simulink model "fftanalyzeri"  (R2012b)
settings: Solver=ode3  SolverMode=SingleTasking  StartTime=0.0  StopTime=20000  RelTol=1e-3
undefined symbols (not defined in the file or in its folder): pfb_coeff_gen_calc
undefined symbols (not defined in the file): fft_bin_flags_, magphmeanmem_, threshmem_
libraries: xbsIndex_r4 x9073, casper_library_misc x119, casper_library_flow_control x51, casper_library_delays x22, xps_library x10
(part 24 of 74)

== system fftanalyzeri/FIFO64_/FIFO32_1/FIFO16Cir_1/CounterArray2/demux16_ ==
  Chan : Inport
  din : Inport  Port=2
  Demux8_ : Subsystem
  Demux8_1 : Subsystem
  Inverter : xbsIndex_r4/Inverter  en=off  latency=0  dbl_ovrd=off  block_type=inv
  lsb_ui3_ : xbsIndex_r4/Slice  nbits=3  boolean_output=off  mode=Lower Bit Location + Width  bit1=0  base1=MSB of Input  bit0=0  base0=LSB of Input  dbl_ovrd=off  block_type=slice
  msb_b_ : xbsIndex_r4/Slice  nbits=1  boolean_output=on  mode=Upper Bit Location + Width  bit1=0  base1=MSB of Input  bit0=0  base0=LSB of Input  dbl_ovrd=off  block_type=slice
  Out1 : Outport
  Out2 : Outport  Port=2
  Out3 : Outport  Port=3
  Out4 : Outport  Port=4
  Out5 : Outport  Port=5
  Out6 : Outport  Port=6
  Out7 : Outport  Port=7
  Out8 : Outport  Port=8
  Out9 : Outport  Port=9
  Out10 : Outport  Port=10
  Out11 : Outport  Port=11
  Out12 : Outport  Port=12
  Out13 : Outport  Port=13
  Out14 : Outport  Port=14
  Out15 : Outport  Port=15
  Out16 : Outport  Port=16
  wires:
  Demux8_1/1(Out0) -> Out9/1
  Demux8_1/6(Out5) -> Out14/1
  Demux8_/5(Out4) -> Out5/1
  Demux8_/7(Out6) -> Out7/1
  Demux8_1/2(Out1) -> Out10/1
  Demux8_1/3(Out2) -> Out11/1
  Demux8_/4(Out3) -> Out4/1
  Demux8_1/7(Out6) -> Out15/1
  Demux8_1/4(Out3) -> Out12/1
  Demux8_/8(Out7) -> Out8/1
  Demux8_/1(Out0) -> Out1/1
  Demux8_1/5(Out4) -> Out13/1
  Demux8_/6(Out5) -> Out6/1
  Demux8_/2(Out1) -> Out2/1
  Demux8_/3(Out2) -> Out3/1
  Demux8_1/8(Out7) -> Out16/1
  Chan/1 -> msb_b_/1, lsb_ui3_/1
  lsb_ui3_/1 -> Demux8_1/1(Addr), Demux8_/1(Addr)
  msb_b_/1 -> Demux8_1/3(en), Inverter/1
  din/1 -> Demux8_1/2(BitIn), Demux8_/2(BitIn)
  Inverter/1 -> Demux8_/3(en)

== system fftanalyzeri/FIFO64_/FIFO32_1/FIFO16Cir_2/CounterArray1/demux16_ ==
  Chan : Inport
  din : Inport  Port=2
  Demux8_ : Subsystem
  Demux8_1 : Subsystem
  Inverter : xbsIndex_r4/Inverter  en=off  latency=0  dbl_ovrd=off  block_type=inv
  lsb_ui3_ : xbsIndex_r4/Slice  nbits=3  boolean_output=off  mode=Lower Bit Location + Width  bit1=0  base1=MSB of Input  bit0=0  base0=LSB of Input  dbl_ovrd=off  block_type=slice
  msb_b_ : xbsIndex_r4/Slice  nbits=1  boolean_output=on  mode=Upper Bit Location + Width  bit1=0  base1=MSB of Input  bit0=0  base0=LSB of Input  dbl_ovrd=off  block_type=slice
  Out1 : Outport
  Out2 : Outport  Port=2
  Out3 : Outport  Port=3
  Out4 : Outport  Port=4
  Out5 : Outport  Port=5
  Out6 : Outport  Port=6
  Out7 : Outport  Port=7
  Out8 : Outport  Port=8
  Out9 : Outport  Port=9
  Out10 : Outport  Port=10
  Out11 : Outport  Port=11
  Out12 : Outport  Port=12
  Out13 : Outport  Port=13
  Out14 : Outport  Port=14
  Out15 : Outport  Port=15
  Out16 : Outport  Port=16
  wires:
  Demux8_1/1(Out0) -> Out9/1
  Demux8_1/6(Out5) -> Out14/1
  Demux8_/5(Out4) -> Out5/1
  Demux8_/7(Out6) -> Out7/1
  Demux8_1/2(Out1) -> Out10/1
  Demux8_1/3(Out2) -> Out11/1
  Demux8_/4(Out3) -> Out4/1
  Demux8_1/7(Out6) -> Out15/1
  Demux8_1/4(Out3) -> Out12/1
  Demux8_/8(Out7) -> Out8/1
  Demux8_/1(Out0) -> Out1/1
  Demux8_1/5(Out4) -> Out13/1
  Demux8_/6(Out5) -> Out6/1
  Demux8_/2(Out1) -> Out2/1
  Demux8_/3(Out2) -> Out3/1
  Demux8_1/8(Out7) -> Out16/1
  Chan/1 -> msb_b_/1, lsb_ui3_/1
  lsb_ui3_/1 -> Demux8_1/1(Addr), Demux8_/1(Addr)
  msb_b_/1 -> Demux8_1/3(en), Inverter/1
  din/1 -> Demux8_1/2(BitIn), Demux8_/2(BitIn)
  Inverter/1 -> Demux8_/3(en)

== system fftanalyzeri/FIFO64_/FIFO32_1/FIFO16Cir_2/CounterArray2/demux16_ ==
  Chan : Inport
  din : Inport  Port=2
  Demux8_ : Subsystem
  Demux8_1 : Subsystem
  Inverter : xbsIndex_r4/Inverter  en=off  latency=0  dbl_ovrd=off  block_type=inv
  lsb_ui3_ : xbsIndex_r4/Slice  nbits=3  boolean_output=off  mode=Lower Bit Location + Width  bit1=0  base1=MSB of Input  bit0=0  base0=LSB of Input  dbl_ovrd=off  block_type=slice
  msb_b_ : xbsIndex_r4/Slice  nbits=1  boolean_output=on  mode=Upper Bit Location + Width  bit1=0  base1=MSB of Input  bit0=0  base0=LSB of Input  dbl_ovrd=off  block_type=slice
  Out1 : Outport
  Out2 : Outport  Port=2
  Out3 : Outport  Port=3
  Out4 : Outport  Port=4
  Out5 : Outport  Port=5
  Out6 : Outport  Port=6
  Out7 : Outport  Port=7
  Out8 : Outport  Port=8
  Out9 : Outport  Port=9
  Out10 : Outport  Port=10
  Out11 : Outport  Port=11
  Out12 : Outport  Port=12
  Out13 : Outport  Port=13
  Out14 : Outport  Port=14
  Out15 : Outport  Port=15
  Out16 : Outport  Port=16
  wires:
  Demux8_1/1(Out0) -> Out9/1
  Demux8_1/6(Out5) -> Out14/1
  Demux8_/5(Out4) -> Out5/1
  Demux8_/7(Out6) -> Out7/1
  Demux8_1/2(Out1) -> Out10/1
  Demux8_1/3(Out2) -> Out11/1
  Demux8_/4(Out3) -> Out4/1
  Demux8_1/7(Out6) -> Out15/1
  Demux8_1/4(Out3) -> Out12/1
  Demux8_/8(Out7) -> Out8/1
  Demux8_/1(Out0) -> Out1/1
  Demux8_1/5(Out4) -> Out13/1
  Demux8_/6(Out5) -> Out6/1
  Demux8_/2(Out1) -> Out2/1
  Demux8_/3(Out2) -> Out3/1
  Demux8_1/8(Out7) -> Out16/1
  Chan/1 -> msb_b_/1, lsb_ui3_/1
  lsb_ui3_/1 -> Demux8_1/1(Addr), Demux8_/1(Addr)
  msb_b_/1 -> Demux8_1/3(en), Inverter/1
  din/1 -> Demux8_1/2(BitIn), Demux8_/2(BitIn)
  Inverter/1 -> Demux8_/3(en)

== system fftanalyzeri/FIFO64_1/FIFO32_0/FIFO16Cir_1/CounterArray1/demux16_ ==
  Chan : Inport
  din : Inport  Port=2
  Demux8_ : Subsystem
  Demux8_1 : Subsystem
  Inverter : xbsIndex_r4/Inverter  en=off  latency=0  dbl_ovrd=off  block_type=inv
  lsb_ui3_ : xbsIndex_r4/Slice  nbits=3  boolean_output=off  mode=Lower Bit Location + Width  bit1=0  base1=MSB of Input  bit0=0  base0=LSB of Input  dbl_ovrd=off  block_type=slice
  msb_b_ : xbsIndex_r4/Slice  nbits=1  boolean_output=on  mode=Upper Bit Location + Width  bit1=0  base1=MSB of Input  bit0=0  base0=LSB of Input  dbl_ovrd=off  block_type=slice
  Out1 : Outport
  Out2 : Outport  Port=2
  Out3 : Outport  Port=3
  Out4 : Outport  Port=4
  Out5 : Outport  Port=5
  Out6 : Outport  Port=6
  Out7 : Outport  Port=7
  Out8 : Outport  Port=8
  Out9 : Outport  Port=9
  Out10 : Outport  Port=10
  Out11 : Outport  Port=11
  Out12 : Outport  Port=12
  Out13 : Outport  Port=13
  Out14 : Outport  Port=14
  Out15 : Outport  Port=15
  Out16 : Outport  Port=16
  wires:
  Demux8_1/1(Out0) -> Out9/1
  Demux8_1/6(Out5) -> Out14/1
  Demux8_/5(Out4) -> Out5/1
  Demux8_/7(Out6) -> Out7/1
  Demux8_1/2(Out1) -> Out10/1
  Demux8_1/3(Out2) -> Out11/1
  Demux8_/4(Out3) -> Out4/1
  Demux8_1/7(Out6) -> Out15/1
  Demux8_1/4(Out3) -> Out12/1
  Demux8_/8(Out7) -> Out8/1
  Demux8_/1(Out0) -> Out1/1
  Demux8_1/5(Out4) -> Out13/1
  Demux8_/6(Out5) -> Out6/1
  Demux8_/2(Out1) -> Out2/1
  Demux8_/3(Out2) -> Out3/1
  Demux8_1/8(Out7) -> Out16/1
  Chan/1 -> msb_b_/1, lsb_ui3_/1
  lsb_ui3_/1 -> Demux8_1/1(Addr), Demux8_/1(Addr)
  msb_b_/1 -> Demux8_1/3(en), Inverter/1
  din/1 -> Demux8_1/2(BitIn), Demux8_/2(BitIn)
  Inverter/1 -> Demux8_/3(en)

== system fftanalyzeri/FIFO64_1/FIFO32_0/FIFO16Cir_1/CounterArray2/demux16_ ==
  Chan : Inport
  din : Inport  Port=2
  Demux8_ : Subsystem
  Demux8_1 : Subsystem
  Inverter : xbsIndex_r4/Inverter  en=off  latency=0  dbl_ovrd=off  block_type=inv
  lsb_ui3_ : xbsIndex_r4/Slice  nbits=3  boolean_output=off  mode=Lower Bit Location + Width  bit1=0  base1=MSB of Input  bit0=0  base0=LSB of Input  dbl_ovrd=off  block_type=slice
  msb_b_ : xbsIndex_r4/Slice  nbits=1  boolean_output=on  mode=Upper Bit Location + Width  bit1=0  base1=MSB of Input  bit0=0  base0=LSB of Input  dbl_ovrd=off  block_type=slice
  Out1 : Outport
  Out2 : Outport  Port=2
  Out3 : Outport  Port=3
  Out4 : Outport  Port=4
  Out5 : Outport  Port=5
  Out6 : Outport  Port=6
  Out7 : Outport  Port=7
  Out8 : Outport  Port=8
  Out9 : Outport  Port=9
  Out10 : Outport  Port=10
  Out11 : Outport  Port=11
  Out12 : Outport  Port=12
  Out13 : Outport  Port=13
  Out14 : Outport  Port=14
  Out15 : Outport  Port=15
  Out16 : Outport  Port=16
  wires:
  Demux8_1/1(Out0) -> Out9/1
  Demux8_1/6(Out5) -> Out14/1
  Demux8_/5(Out4) -> Out5/1
  Demux8_/7(Out6) -> Out7/1
  Demux8_1/2(Out1) -> Out10/1
  Demux8_1/3(Out2) -> Out11/1
  Demux8_/4(Out3) -> Out4/1
  Demux8_1/7(Out6) -> Out15/1
  Demux8_1/4(Out3) -> Out12/1
  Demux8_/8(Out7) -> Out8/1
  Demux8_/1(Out0) -> Out1/1
  Demux8_1/5(Out4) -> Out13/1
  Demux8_/6(Out5) -> Out6/1
  Demux8_/2(Out1) -> Out2/1
  Demux8_/3(Out2) -> Out3/1
  Demux8_1/8(Out7) -> Out16/1
  Chan/1 -> msb_b_/1, lsb_ui3_/1
  lsb_ui3_/1 -> Demux8_1/1(Addr), Demux8_/1(Addr)
  msb_b_/1 -> Demux8_1/3(en), Inverter/1
  din/1 -> Demux8_1/2(BitIn), Demux8_/2(BitIn)
  Inverter/1 -> Demux8_/3(en)

== system fftanalyzeri/FIFO64_1/FIFO32_0/FIFO16Cir_2/CounterArray1/demux16_ ==
  Chan : Inport
  din : Inport  Port=2
  Demux8_ : Subsystem
  Demux8_1 : Subsystem
  Inverter : xbsIndex_r4/Inverter  en=off  latency=0  dbl_ovrd=off  block_type=inv
  lsb_ui3_ : xbsIndex_r4/Slice  nbits=3  boolean_output=off  mode=Lower Bit Location + Width  bit1=0  base1=MSB of Input  bit0=0  base0=LSB of Input  dbl_ovrd=off  block_type=slice
  msb_b_ : xbsIndex_r4/Slice  nbits=1  boolean_output=on  mode=Upper Bit Location + Width  bit1=0  base1=MSB of Input  bit0=0  base0=LSB of Input  dbl_ovrd=off  block_type=slice
  Out1 : Outport
  Out2 : Outport  Port=2
  Out3 : Outport  Port=3
  Out4 : Outport  Port=4
  Out5 : Outport  Port=5
  Out6 : Outport  Port=6
  Out7 : Outport  Port=7
  Out8 : Outport  Port=8
  Out9 : Outport  Port=9
  Out10 : Outport  Port=10
  Out11 : Outport  Port=11
  Out12 : Outport  Port=12
  Out13 : Outport  Port=13
  Out14 : Outport  Port=14
  Out15 : Outport  Port=15
  Out16 : Outport  Port=16
  wires:
  Demux8_1/1(Out0) -> Out9/1
  Demux8_1/6(Out5) -> Out14/1
  Demux8_/5(Out4) -> Out5/1
  Demux8_/7(Out6) -> Out7/1
  Demux8_1/2(Out1) -> Out10/1
  Demux8_1/3(Out2) -> Out11/1
  Demux8_/4(Out3) -> Out4/1
  Demux8_1/7(Out6) -> Out15/1
  Demux8_1/4(Out3) -> Out12/1
  Demux8_/8(Out7) -> Out8/1
  Demux8_/1(Out0) -> Out1/1
  Demux8_1/5(Out4) -> Out13/1
  Demux8_/6(Out5) -> Out6/1
  Demux8_/2(Out1) -> Out2/1
  Demux8_/3(Out2) -> Out3/1
  Demux8_1/8(Out7) -> Out16/1
  Chan/1 -> msb_b_/1, lsb_ui3_/1
  lsb_ui3_/1 -> Demux8_1/1(Addr), Demux8_/1(Addr)
  msb_b_/1 -> Demux8_1/3(en), Inverter/1
  din/1 -> Demux8_1/2(BitIn), Demux8_/2(BitIn)
  Inverter/1 -> Demux8_/3(en)

== system fftanalyzeri/FIFO64_1/FIFO32_0/FIFO16Cir_2/CounterArray2/demux16_ ==
  Chan : Inport
  din : Inport  Port=2
  Demux8_ : Subsystem
  Demux8_1 : Subsystem
  Inverter : xbsIndex_r4/Inverter  en=off  latency=0  dbl_ovrd=off  block_type=inv
  lsb_ui3_ : xbsIndex_r4/Slice  nbits=3  boolean_output=off  mode=Lower Bit Location + Width  bit1=0  base1=MSB of Input  bit0=0  base0=LSB of Input  dbl_ovrd=off  block_type=slice
  msb_b_ : xbsIndex_r4/Slice  nbits=1  boolean_output=on  mode=Upper Bit Location + Width  bit1=0  base1=MSB of Input  bit0=0  base0=LSB of Input  dbl_ovrd=off  block_type=slice
  Out1 : Outport
  Out2 : Outport  Port=2
  Out3 : Outport  Port=3
  Out4 : Outport  Port=4
  Out5 : Outport  Port=5
  Out6 : Outport  Port=6
  Out7 : Outport  Port=7
  Out8 : Outport  Port=8
  Out9 : Outport  Port=9
  Out10 : Outport  Port=10
  Out11 : Outport  Port=11
  Out12 : Outport  Port=12
  Out13 : Outport  Port=13
  Out14 : Outport  Port=14
  Out15 : Outport  Port=15
  Out16 : Outport  Port=16
  wires:
  Demux8_1/1(Out0) -> Out9/1
  Demux8_1/6(Out5) -> Out14/1
  Demux8_/5(Out4) -> Out5/1
  Demux8_/7(Out6) -> Out7/1
  Demux8_1/2(Out1) -> Out10/1
  Demux8_1/3(Out2) -> Out11/1
  Demux8_/4(Out3) -> Out4/1
  Demux8_1/7(Out6) -> Out15/1
  Demux8_1/4(Out3) -> Out12/1
  Demux8_/8(Out7) -> Out8/1
  Demux8_/1(Out0) -> Out1/1
  Demux8_1/5(Out4) -> Out13/1
  Demux8_/6(Out5) -> Out6/1
  Demux8_/2(Out1) -> Out2/1
  Demux8_/3(Out2) -> Out3/1
  Demux8_1/8(Out7) -> Out16/1
  Chan/1 -> msb_b_/1, lsb_ui3_/1
  lsb_ui3_/1 -> Demux8_1/1(Addr), Demux8_/1(Addr)
  msb_b_/1 -> Demux8_1/3(en), Inverter/1
  din/1 -> Demux8_1/2(BitIn), Demux8_/2(BitIn)
  Inverter/1 -> Demux8_/3(en)

== system fftanalyzeri/FIFO64_1/FIFO32_1/FIFO16Cir_1/CounterArray1/demux16_ ==
  Chan : Inport
  din : Inport  Port=2
  Demux8_ : Subsystem
  Demux8_1 : Subsystem
  Inverter : xbsIndex_r4/Inverter  en=off  latency=0  dbl_ovrd=off  block_type=inv
  lsb_ui3_ : xbsIndex_r4/Slice  nbits=3  boolean_output=off  mode=Lower Bit Location + Width  bit1=0  base1=MSB of Input  bit0=0  base0=LSB of Input  dbl_ovrd=off  block_type=slice
  msb_b_ : xbsIndex_r4/Slice  nbits=1  boolean_output=on  mode=Upper Bit Location + Width  bit1=0  base1=MSB of Input  bit0=0  base0=LSB of Input  dbl_ovrd=off  block_type=slice
  Out1 : Outport
  Out2 : Outport  Port=2
  Out3 : Outport  Port=3
  Out4 : Outport  Port=4
  Out5 : Outport  Port=5
  Out6 : Outport  Port=6
  Out7 : Outport  Port=7
  Out8 : Outport  Port=8
  Out9 : Outport  Port=9
  Out10 : Outport  Port=10
  Out11 : Outport  Port=11
  Out12 : Outport  Port=12
  Out13 : Outport  Port=13
  Out14 : Outport  Port=14
  Out15 : Outport  Port=15
  Out16 : Outport  Port=16
  wires:
  Demux8_1/1(Out0) -> Out9/1
  Demux8_1/6(Out5) -> Out14/1
  Demux8_/5(Out4) -> Out5/1
  Demux8_/7(Out6) -> Out7/1
  Demux8_1/2(Out1) -> Out10/1
  Demux8_1/3(Out2) -> Out11/1
  Demux8_/4(Out3) -> Out4/1
  Demux8_1/7(Out6) -> Out15/1
  Demux8_1/4(Out3) -> Out12/1
  Demux8_/8(Out7) -> Out8/1
  Demux8_/1(Out0) -> Out1/1
  Demux8_1/5(Out4) -> Out13/1
  Demux8_/6(Out5) -> Out6/1
  Demux8_/2(Out1) -> Out2/1
  Demux8_/3(Out2) -> Out3/1
  Demux8_1/8(Out7) -> Out16/1
  Chan/1 -> msb_b_/1, lsb_ui3_/1
  lsb_ui3_/1 -> Demux8_1/1(Addr), Demux8_/1(Addr)
  msb_b_/1 -> Demux8_1/3(en), Inverter/1
  din/1 -> Demux8_1/2(BitIn), Demux8_/2(BitIn)
  Inverter/1 -> Demux8_/3(en)

== system fftanalyzeri/FIFO64_1/FIFO32_1/FIFO16Cir_1/CounterArray2/demux16_ ==
  Chan : Inport
  din : Inport  Port=2
  Demux8_ : Subsystem
  Demux8_1 : Subsystem
  Inverter : xbsIndex_r4/Inverter  en=off  latency=0  dbl_ovrd=off  block_type=inv
  lsb_ui3_ : xbsIndex_r4/Slice  nbits=3  boolean_output=off  mode=Lower Bit Location + Width  bit1=0  base1=MSB of Input  bit0=0  base0=LSB of Input  dbl_ovrd=off  block_type=slice
  msb_b_ : xbsIndex_r4/Slice  nbits=1  boolean_output=on  mode=Upper Bit Location + Width  bit1=0  base1=MSB of Input  bit0=0  base0=LSB of Input  dbl_ovrd=off  block_type=slice
  Out1 : Outport
  Out2 : Outport  Port=2
  Out3 : Outport  Port=3
  Out4 : Outport  Port=4
  Out5 : Outport  Port=5
  Out6 : Outport  Port=6
  Out7 : Outport  Port=7
  Out8 : Outport  Port=8
  Out9 : Outport  Port=9
  Out10 : Outport  Port=10
  Out11 : Outport  Port=11
  Out12 : Outport  Port=12
  Out13 : Outport  Port=13
  Out14 : Outport  Port=14
  Out15 : Outport  Port=15
  Out16 : Outport  Port=16
  wires:
  Demux8_1/1(Out0) -> Out9/1
  Demux8_1/6(Out5) -> Out14/1
  Demux8_/5(Out4) -> Out5/1
  Demux8_/7(Out6) -> Out7/1
  Demux8_1/2(Out1) -> Out10/1
  Demux8_1/3(Out2) -> Out11/1
  Demux8_/4(Out3) -> Out4/1
  Demux8_1/7(Out6) -> Out15/1
  Demux8_1/4(Out3) -> Out12/1
  Demux8_/8(Out7) -> Out8/1
  Demux8_/1(Out0) -> Out1/1
  Demux8_1/5(Out4) -> Out13/1
  Demux8_/6(Out5) -> Out6/1
  Demux8_/2(Out1) -> Out2/1
  Demux8_/3(Out2) -> Out3/1
  Demux8_1/8(Out7) -> Out16/1
  Chan/1 -> msb_b_/1, lsb_ui3_/1
  lsb_ui3_/1 -> Demux8_1/1(Addr), Demux8_/1(Addr)
  msb_b_/1 -> Demux8_1/3(en), Inverter/1
  din/1 -> Demux8_1/2(BitIn), Demux8_/2(BitIn)
  Inverter/1 -> Demux8_/3(en)

== system fftanalyzeri/FIFO64_1/FIFO32_1/FIFO16Cir_2/CounterArray1/demux16_ ==
  Chan : Inport
  din : Inport  Port=2
  Demux8_ : Subsystem
  Demux8_1 : Subsystem
  Inverter : xbsIndex_r4/Inverter  en=off  latency=0  dbl_ovrd=off  block_type=inv
  lsb_ui3_ : xbsIndex_r4/Slice  nbits=3  boolean_output=off  mode=Lower Bit Location + Width  bit1=0  base1=MSB of Input  bit0=0  base0=LSB of Input  dbl_ovrd=off  block_type=slice
  msb_b_ : xbsIndex_r4/Slice  nbits=1  boolean_output=on  mode=Upper Bit Location + Width  bit1=0  base1=MSB of Input  bit0=0  base0=LSB of Input  dbl_ovrd=off  block_type=slice
  Out1 : Outport
  Out2 : Outport  Port=2
  Out3 : Outport  Port=3
  Out4 : Outport  Port=4
  Out5 : Outport  Port=5
  Out6 : Outport  Port=6
  Out7 : Outport  Port=7
  Out8 : Outport  Port=8
  Out9 : Outport  Port=9
  Out10 : Outport  Port=10
  Out11 : Outport  Port=11
  Out12 : Outport  Port=12
  Out13 : Outport  Port=13
  Out14 : Outport  Port=14
  Out15 : Outport  Port=15
  Out16 : Outport  Port=16
  wires:
  Demux8_1/1(Out0) -> Out9/1
  Demux8_1/6(Out5) -> Out14/1
  Demux8_/5(Out4) -> Out5/1
  Demux8_/7(Out6) -> Out7/1
  Demux8_1/2(Out1) -> Out10/1
  Demux8_1/3(Out2) -> Out11/1
  Demux8_/4(Out3) -> Out4/1
  Demux8_1/7(Out6) -> Out15/1
  Demux8_1/4(Out3) -> Out12/1
  Demux8_/8(Out7) -> Out8/1
  Demux8_/1(Out0) -> Out1/1
  Demux8_1/5(Out4) -> Out13/1
  Demux8_/6(Out5) -> Out6/1
  Demux8_/2(Out1) -> Out2/1
  Demux8_/3(Out2) -> Out3/1
  Demux8_1/8(Out7) -> Out16/1
  Chan/1 -> msb_b_/1, lsb_ui3_/1
  lsb_ui3_/1 -> Demux8_1/1(Addr), Demux8_/1(Addr)
  msb_b_/1 -> Demux8_1/3(en), Inverter/1
  din/1 -> Demux8_1/2(BitIn), Demux8_/2(BitIn)
  Inverter/1 -> Demux8_/3(en)

== system fftanalyzeri/FIFO64_1/FIFO32_1/FIFO16Cir_2/CounterArray2/demux16_ ==
  Chan : Inport
  din : Inport  Port=2
  Demux8_ : Subsystem
  Demux8_1 : Subsystem
  Inverter : xbsIndex_r4/Inverter  en=off  latency=0  dbl_ovrd=off  block_type=inv
  lsb_ui3_ : xbsIndex_r4/Slice  nbits=3  boolean_output=off  mode=Lower Bit Location + Width  bit1=0  base1=MSB of Input  bit0=0  base0=LSB of Input  dbl_ovrd=off  block_type=slice
  msb_b_ : xbsIndex_r4/Slice  nbits=1  boolean_output=on  mode=Upper Bit Location + Width  bit1=0  base1=MSB of Input  bit0=0  base0=LSB of Input  dbl_ovrd=off  block_type=slice
  Out1 : Outport
  Out2 : Outport  Port=2
  Out3 : Outport  Port=3
  Out4 : Outport  Port=4
  Out5 : Outport  Port=5
  Out6 : Outport  Port=6
  Out7 : Outport  Port=7
  Out8 : Outport  Port=8
  Out9 : Outport  Port=9
  Out10 : Outport  Port=10
  Out11 : Outport  Port=11
  Out12 : Outport  Port=12
  Out13 : Outport  Port=13
  Out14 : Outport  Port=14
  Out15 : Outport  Port=15
  Out16 : Outport  Port=16
  wires:
  Demux8_1/1(Out0) -> Out9/1
  Demux8_1/6(Out5) -> Out14/1
  Demux8_/5(Out4) -> Out5/1
  Demux8_/7(Out6) -> Out7/1
  Demux8_1/2(Out1) -> Out10/1
  Demux8_1/3(Out2) -> Out11/1
  Demux8_/4(Out3) -> Out4/1
  Demux8_1/7(Out6) -> Out15/1
  Demux8_1/4(Out3) -> Out12/1
  Demux8_/8(Out7) -> Out8/1
  Demux8_/1(Out0) -> Out1/1
  Demux8_1/5(Out4) -> Out13/1
  Demux8_/6(Out5) -> Out6/1
  Demux8_/2(Out1) -> Out2/1
  Demux8_/3(Out2) -> Out3/1
  Demux8_1/8(Out7) -> Out16/1
  Chan/1 -> msb_b_/1, lsb_ui3_/1
  lsb_ui3_/1 -> Demux8_1/1(Addr), Demux8_/1(Addr)
  msb_b_/1 -> Demux8_1/3(en), Inverter/1
  din/1 -> Demux8_1/2(BitIn), Demux8_/2(BitIn)
  Inverter/1 -> Demux8_/3(en)

== system fftanalyzeri/FIFO64_2/FIFO32_0/FIFO16Cir_1/CounterArray1/demux16_ ==
  Chan : Inport
  din : Inport  Port=2
  Demux8_ : Subsystem
  Demux8_1 : Subsystem
  Inverter : xbsIndex_r4/Inverter  en=off  latency=0  dbl_ovrd=off  block_type=inv
  lsb_ui3_ : xbsIndex_r4/Slice  nbits=3  boolean_output=off  mode=Lower Bit Location + Width  bit1=0  base1=MSB of Input  bit0=0  base0=LSB of Input  dbl_ovrd=off  block_type=slice
  msb_b_ : xbsIndex_r4/Slice  nbits=1  boolean_output=on  mode=Upper Bit Location + Width  bit1=0  base1=MSB of Input  bit0=0  base0=LSB of Input  dbl_ovrd=off  block_type=slice
  Out1 : Outport
  Out2 : Outport  Port=2
  Out3 : Outport  Port=3
  Out4 : Outport  Port=4
  Out5 : Outport  Port=5
  Out6 : Outport  Port=6
  Out7 : Outport  Port=7
  Out8 : Outport  Port=8
  Out9 : Outport  Port=9
  Out10 : Outport  Port=10
  Out11 : Outport  Port=11
  Out12 : Outport  Port=12
  Out13 : Outport  Port=13
  Out14 : Outport  Port=14
  Out15 : Outport  Port=15
  Out16 : Outport  Port=16
  wires:
  Demux8_1/1(Out0) -> Out9/1
  Demux8_1/6(Out5) -> Out14/1
  Demux8_/5(Out4) -> Out5/1
  Demux8_/7(Out6) -> Out7/1
  Demux8_1/2(Out1) -> Out10/1
  Demux8_1/3(Out2) -> Out11/1
  Demux8_/4(Out3) -> Out4/1
  Demux8_1/7(Out6) -> Out15/1
  Demux8_1/4(Out3) -> Out12/1
  Demux8_/8(Out7) -> Out8/1
  Demux8_/1(Out0) -> Out1/1
  Demux8_1/5(Out4) -> Out13/1
  Demux8_/6(Out5) -> Out6/1
  Demux8_/2(Out1) -> Out2/1
  Demux8_/3(Out2) -> Out3/1
  Demux8_1/8(Out7) -> Out16/1
  Chan/1 -> msb_b_/1, lsb_ui3_/1
  lsb_ui3_/1 -> Demux8_1/1(Addr), Demux8_/1(Addr)
  msb_b_/1 -> Demux8_1/3(en), Inverter/1
  din/1 -> Demux8_1/2(BitIn), Demux8_/2(BitIn)
  Inverter/1 -> Demux8_/3(en)

== system fftanalyzeri/FIFO64_2/FIFO32_0/FIFO16Cir_1/CounterArray2/demux16_ ==
  Chan : Inport
  din : Inport  Port=2
  Demux8_ : Subsystem
  Demux8_1 : Subsystem
  Inverter : xbsIndex_r4/Inverter  en=off  latency=0  dbl_ovrd=off  block_type=inv
  lsb_ui3_ : xbsIndex_r4/Slice  nbits=3  boolean_output=off  mode=Lower Bit Location + Width  bit1=0  base1=MSB of Input  bit0=0  base0=LSB of Input  dbl_ovrd=off  block_type=slice
  msb_b_ : xbsIndex_r4/Slice  nbits=1  boolean_output=on  mode=Upper Bit Location + Width  bit1=0  base1=MSB of Input  bit0=0  base0=LSB of Input  dbl_ovrd=off  block_type=slice
  Out1 : Outport
  Out2 : Outport  Port=2
  Out3 : Outport  Port=3
  Out4 : Outport  Port=4
  Out5 : Outport  Port=5
  Out6 : Outport  Port=6
  Out7 : Outport  Port=7
  Out8 : Outport  Port=8
  Out9 : Outport  Port=9
  Out10 : Outport  Port=10
  Out11 : Outport  Port=11
  Out12 : Outport  Port=12
  Out13 : Outport  Port=13
  Out14 : Outport  Port=14
  Out15 : Outport  Port=15
  Out16 : Outport  Port=16
  wires:
  Demux8_1/1(Out0) -> Out9/1
  Demux8_1/6(Out5) -> Out14/1
  Demux8_/5(Out4) -> Out5/1
  Demux8_/7(Out6) -> Out7/1
  Demux8_1/2(Out1) -> Out10/1
  Demux8_1/3(Out2) -> Out11/1
  Demux8_/4(Out3) -> Out4/1
  Demux8_1/7(Out6) -> Out15/1
  Demux8_1/4(Out3) -> Out12/1
  Demux8_/8(Out7) -> Out8/1
  Demux8_/1(Out0) -> Out1/1
  Demux8_1/5(Out4) -> Out13/1
  Demux8_/6(Out5) -> Out6/1
  Demux8_/2(Out1) -> Out2/1
  Demux8_/3(Out2) -> Out3/1
  Demux8_1/8(Out7) -> Out16/1
  Chan/1 -> msb_b_/1, lsb_ui3_/1
  lsb_ui3_/1 -> Demux8_1/1(Addr), Demux8_/1(Addr)
  msb_b_/1 -> Demux8_1/3(en), Inverter/1
  din/1 -> Demux8_1/2(BitIn), Demux8_/2(BitIn)
  Inverter/1 -> Demux8_/3(en)

== system fftanalyzeri/FIFO64_2/FIFO32_0/FIFO16Cir_2/CounterArray1/demux16_ ==
  Chan : Inport
  din : Inport  Port=2
  Demux8_ : Subsystem
  Demux8_1 : Subsystem
  Inverter : xbsIndex_r4/Inverter  en=off  latency=0  dbl_ovrd=off  block_type=inv
  lsb_ui3_ : xbsIndex_r4/Slice  nbits=3  boolean_output=off  mode=Lower Bit Location + Width  bit1=0  base1=MSB of Input  bit0=0  base0=LSB of Input  dbl_ovrd=off  block_type=slice
  msb_b_ : xbsIndex_r4/Slice  nbits=1  boolean_output=on  mode=Upper Bit Location + Width  bit1=0  base1=MSB of Input  bit0=0  base0=LSB of Input  dbl_ovrd=off  block_type=slice
  Out1 : Outport
  Out2 : Outport  Port=2
  Out3 : Outport  Port=3
  Out4 : Outport  Port=4
  Out5 : Outport  Port=5
  Out6 : Outport  Port=6
  Out7 : Outport  Port=7
  Out8 : Outport  Port=8
  Out9 : Outport  Port=9
  Out10 : Outport  Port=10
  Out11 : Outport  Port=11
  Out12 : Outport  Port=12
  Out13 : Outport  Port=13
  Out14 : Outport  Port=14
  Out15 : Outport  Port=15
  Out16 : Outport  Port=16
  wires:
  Demux8_1/1(Out0) -> Out9/1
  Demux8_1/6(Out5) -> Out14/1
  Demux8_/5(Out4) -> Out5/1
  Demux8_/7(Out6) -> Out7/1
  Demux8_1/2(Out1) -> Out10/1
  Demux8_1/3(Out2) -> Out11/1
  Demux8_/4(Out3) -> Out4/1
  Demux8_1/7(Out6) -> Out15/1
  Demux8_1/4(Out3) -> Out12/1
  Demux8_/8(Out7) -> Out8/1
  Demux8_/1(Out0) -> Out1/1
  Demux8_1/5(Out4) -> Out13/1
  Demux8_/6(Out5) -> Out6/1
  Demux8_/2(Out1) -> Out2/1
  Demux8_/3(Out2) -> Out3/1
  Demux8_1/8(Out7) -> Out16/1
  Chan/1 -> msb_b_/1, lsb_ui3_/1
  lsb_ui3_/1 -> Demux8_1/1(Addr), Demux8_/1(Addr)
  msb_b_/1 -> Demux8_1/3(en), Inverter/1
  din/1 -> Demux8_1/2(BitIn), Demux8_/2(BitIn)
  Inverter/1 -> Demux8_/3(en)

== system fftanalyzeri/FIFO64_2/FIFO32_0/FIFO16Cir_2/CounterArray2/demux16_ ==
  Chan : Inport
  din : Inport  Port=2
  Demux8_ : Subsystem
  Demux8_1 : Subsystem
  Inverter : xbsIndex_r4/Inverter  en=off  latency=0  dbl_ovrd=off  block_type=inv
  lsb_ui3_ : xbsIndex_r4/Slice  nbits=3  boolean_output=off  mode=Lower Bit Location + Width  bit1=0  base1=MSB of Input  bit0=0  base0=LSB of Input  dbl_ovrd=off  block_type=slice
  msb_b_ : xbsIndex_r4/Slice  nbits=1  boolean_output=on  mode=Upper Bit Location + Width  bit1=0  base1=MSB of Input  bit0=0  base0=LSB of Input  dbl_ovrd=off  block_type=slice
  Out1 : Outport
  Out2 : Outport  Port=2
  Out3 : Outport  Port=3
  Out4 : Outport  Port=4
  Out5 : Outport  Port=5
  Out6 : Outport  Port=6
  Out7 : Outport  Port=7
  Out8 : Outport  Port=8
  Out9 : Outport  Port=9
  Out10 : Outport  Port=10
  Out11 : Outport  Port=11
  Out12 : Outport  Port=12
  Out13 : Outport  Port=13
  Out14 : Outport  Port=14
  Out15 : Outport  Port=15
  Out16 : Outport  Port=16
  wires:
  Demux8_1/1(Out0) -> Out9/1
  Demux8_1/6(Out5) -> Out14/1
  Demux8_/5(Out4) -> Out5/1
  Demux8_/7(Out6) -> Out7/1
  Demux8_1/2(Out1) -> Out10/1
  Demux8_1/3(Out2) -> Out11/1
  Demux8_/4(Out3) -> Out4/1
  Demux8_1/7(Out6) -> Out15/1
  Demux8_1/4(Out3) -> Out12/1
  Demux8_/8(Out7) -> Out8/1
  Demux8_/1(Out0) -> Out1/1
  Demux8_1/5(Out4) -> Out13/1
  Demux8_/6(Out5) -> Out6/1
  Demux8_/2(Out1) -> Out2/1
  Demux8_/3(Out2) -> Out3/1
  Demux8_1/8(Out7) -> Out16/1
  Chan/1 -> msb_b_/1, lsb_ui3_/1
  lsb_ui3_/1 -> Demux8_1/1(Addr), Demux8_/1(Addr)
  msb_b_/1 -> Demux8_1/3(en), Inverter/1
  din/1 -> Demux8_1/2(BitIn), Demux8_/2(BitIn)
  Inverter/1 -> Demux8_/3(en)

== system fftanalyzeri/FIFO64_2/FIFO32_1/FIFO16Cir_1/CounterArray1/demux16_ ==
  Chan : Inport
  din : Inport  Port=2
  Demux8_ : Subsystem
  Demux8_1 : Subsystem
  Inverter : xbsIndex_r4/Inverter  en=off  latency=0  dbl_ovrd=off  block_type=inv
  lsb_ui3_ : xbsIndex_r4/Slice  nbits=3  boolean_output=off  mode=Lower Bit Location + Width  bit1=0  base1=MSB of Input  bit0=0  base0=LSB of Input  dbl_ovrd=off  block_type=slice
  msb_b_ : xbsIndex_r4/Slice  nbits=1  boolean_output=on  mode=Upper Bit Location + Width  bit1=0  base1=MSB of Input  bit0=0  base0=LSB of Input  dbl_ovrd=off  block_type=slice
  Out1 : Outport
  Out2 : Outport  Port=2
  Out3 : Outport  Port=3
  Out4 : Outport  Port=4
  Out5 : Outport  Port=5
  Out6 : Outport  Port=6
  Out7 : Outport  Port=7
  Out8 : Outport  Port=8
  Out9 : Outport  Port=9
  Out10 : Outport  Port=10
  Out11 : Outport  Port=11
  Out12 : Outport  Port=12
  Out13 : Outport  Port=13
  Out14 : Outport  Port=14
  Out15 : Outport  Port=15
  Out16 : Outport  Port=16
  wires:
  Demux8_1/1(Out0) -> Out9/1
  Demux8_1/6(Out5) -> Out14/1
  Demux8_/5(Out4) -> Out5/1
  Demux8_/7(Out6) -> Out7/1
  Demux8_1/2(Out1) -> Out10/1
  Demux8_1/3(Out2) -> Out11/1
  Demux8_/4(Out3) -> Out4/1
  Demux8_1/7(Out6) -> Out15/1
  Demux8_1/4(Out3) -> Out12/1
  Demux8_/8(Out7) -> Out8/1
  Demux8_/1(Out0) -> Out1/1
  Demux8_1/5(Out4) -> Out13/1
  Demux8_/6(Out5) -> Out6/1
  Demux8_/2(Out1) -> Out2/1
  Demux8_/3(Out2) -> Out3/1
  Demux8_1/8(Out7) -> Out16/1
  Chan/1 -> msb_b_/1, lsb_ui3_/1
  lsb_ui3_/1 -> Demux8_1/1(Addr), Demux8_/1(Addr)
  msb_b_/1 -> Demux8_1/3(en), Inverter/1
  din/1 -> Demux8_1/2(BitIn), Demux8_/2(BitIn)
  Inverter/1 -> Demux8_/3(en)

== system fftanalyzeri/FIFO64_2/FIFO32_1/FIFO16Cir_1/CounterArray2/demux16_ ==
  Chan : Inport
  din : Inport  Port=2
  Demux8_ : Subsystem
  Demux8_1 : Subsystem
  Inverter : xbsIndex_r4/Inverter  en=off  latency=0  dbl_ovrd=off  block_type=inv
  lsb_ui3_ : xbsIndex_r4/Slice  nbits=3  boolean_output=off  mode=Lower Bit Location + Width  bit1=0  base1=MSB of Input  bit0=0  base0=LSB of Input  dbl_ovrd=off  block_type=slice
  msb_b_ : xbsIndex_r4/Slice  nbits=1  boolean_output=on  mode=Upper Bit Location + Width  bit1=0  base1=MSB of Input  bit0=0  base0=LSB of Input  dbl_ovrd=off  block_type=slice
  Out1 : Outport
  Out2 : Outport  Port=2
  Out3 : Outport  Port=3
  Out4 : Outport  Port=4
  Out5 : Outport  Port=5
  Out6 : Outport  Port=6
  Out7 : Outport  Port=7
  Out8 : Outport  Port=8
  Out9 : Outport  Port=9
  Out10 : Outport  Port=10
  Out11 : Outport  Port=11
  Out12 : Outport  Port=12
  Out13 : Outport  Port=13
  Out14 : Outport  Port=14
  Out15 : Outport  Port=15
  Out16 : Outport  Port=16
  wires:
  Demux8_1/1(Out0) -> Out9/1
  Demux8_1/6(Out5) -> Out14/1
  Demux8_/5(Out4) -> Out5/1
  Demux8_/7(Out6) -> Out7/1
  Demux8_1/2(Out1) -> Out10/1
  Demux8_1/3(Out2) -> Out11/1
  Demux8_/4(Out3) -> Out4/1
  Demux8_1/7(Out6) -> Out15/1
  Demux8_1/4(Out3) -> Out12/1
  Demux8_/8(Out7) -> Out8/1
  Demux8_/1(Out0) -> Out1/1
  Demux8_1/5(Out4) -> Out13/1
  Demux8_/6(Out5) -> Out6/1
  Demux8_/2(Out1) -> Out2/1
  Demux8_/3(Out2) -> Out3/1
  Demux8_1/8(Out7) -> Out16/1
  Chan/1 -> msb_b_/1, lsb_ui3_/1
  lsb_ui3_/1 -> Demux8_1/1(Addr), Demux8_/1(Addr)
  msb_b_/1 -> Demux8_1/3(en), Inverter/1
  din/1 -> Demux8_1/2(BitIn), Demux8_/2(BitIn)
  Inverter/1 -> Demux8_/3(en)

== system fftanalyzeri/FIFO64_2/FIFO32_1/FIFO16Cir_2/CounterArray1/demux16_ ==
  Chan : Inport
  din : Inport  Port=2
  Demux8_ : Subsystem
  Demux8_1 : Subsystem
  Inverter : xbsIndex_r4/Inverter  en=off  latency=0  dbl_ovrd=off  block_type=inv
  lsb_ui3_ : xbsIndex_r4/Slice  nbits=3  boolean_output=off  mode=Lower Bit Location + Width  bit1=0  base1=MSB of Input  bit0=0  base0=LSB of Input  dbl_ovrd=off  block_type=slice
  msb_b_ : xbsIndex_r4/Slice  nbits=1  boolean_output=on  mode=Upper Bit Location + Width  bit1=0  base1=MSB of Input  bit0=0  base0=LSB of Input  dbl_ovrd=off  block_type=slice
  Out1 : Outport
  Out2 : Outport  Port=2
  Out3 : Outport  Port=3
  Out4 : Outport  Port=4
  Out5 : Outport  Port=5
  Out6 : Outport  Port=6
  Out7 : Outport  Port=7
  Out8 : Outport  Port=8
  Out9 : Outport  Port=9
  Out10 : Outport  Port=10
  Out11 : Outport  Port=11
  Out12 : Outport  Port=12
  Out13 : Outport  Port=13
  Out14 : Outport  Port=14
  Out15 : Outport  Port=15
  Out16 : Outport  Port=16
  wires:
  Demux8_1/1(Out0) -> Out9/1
  Demux8_1/6(Out5) -> Out14/1
  Demux8_/5(Out4) -> Out5/1
  Demux8_/7(Out6) -> Out7/1
  Demux8_1/2(Out1) -> Out10/1
  Demux8_1/3(Out2) -> Out11/1
  Demux8_/4(Out3) -> Out4/1
  Demux8_1/7(Out6) -> Out15/1
  Demux8_1/4(Out3) -> Out12/1
  Demux8_/8(Out7) -> Out8/1
  Demux8_/1(Out0) -> Out1/1
  Demux8_1/5(Out4) -> Out13/1
  Demux8_/6(Out5) -> Out6/1
  Demux8_/2(Out1) -> Out2/1
  Demux8_/3(Out2) -> Out3/1
  Demux8_1/8(Out7) -> Out16/1
  Chan/1 -> msb_b_/1, lsb_ui3_/1
  lsb_ui3_/1 -> Demux8_1/1(Addr), Demux8_/1(Addr)
  msb_b_/1 -> Demux8_1/3(en), Inverter/1
  din/1 -> Demux8_1/2(BitIn), Demux8_/2(BitIn)
  Inverter/1 -> Demux8_/3(en)

== system fftanalyzeri/FIFO64_2/FIFO32_1/FIFO16Cir_2/CounterArray2/demux16_ ==
  Chan : Inport
  din : Inport  Port=2
  Demux8_ : Subsystem
  Demux8_1 : Subsystem
  Inverter : xbsIndex_r4/Inverter  en=off  latency=0  dbl_ovrd=off  block_type=inv
  lsb_ui3_ : xbsIndex_r4/Slice  nbits=3  boolean_output=off  mode=Lower Bit Location + Width  bit1=0  base1=MSB of Input  bit0=0  base0=LSB of Input  dbl_ovrd=off  block_type=slice
  msb_b_ : xbsIndex_r4/Slice  nbits=1  boolean_output=on  mode=Upper Bit Location + Width  bit1=0  base1=MSB of Input  bit0=0  base0=LSB of Input  dbl_ovrd=off  block_type=slice
  Out1 : Outport
  Out2 : Outport  Port=2
  Out3 : Outport  Port=3
  Out4 : Outport  Port=4
  Out5 : Outport  Port=5
  Out6 : Outport  Port=6
  Out7 : Outport  Port=7
  Out8 : Outport  Port=8
  Out9 : Outport  Port=9
  Out10 : Outport  Port=10
  Out11 : Outport  Port=11
  Out12 : Outport  Port=12
  Out13 : Outport  Port=13
  Out14 : Outport  Port=14
  Out15 : Outport  Port=15
  Out16 : Outport  Port=16
  wires:
  Demux8_1/1(Out0) -> Out9/1
  Demux8_1/6(Out5) -> Out14/1
  Demux8_/5(Out4) -> Out5/1
  Demux8_/7(Out6) -> Out7/1
  Demux8_1/2(Out1) -> Out10/1
  Demux8_1/3(Out2) -> Out11/1
  Demux8_/4(Out3) -> Out4/1
  Demux8_1/7(Out6) -> Out15/1
  Demux8_1/4(Out3) -> Out12/1
  Demux8_/8(Out7) -> Out8/1
  Demux8_/1(Out0) -> Out1/1
  Demux8_1/5(Out4) -> Out13/1
  Demux8_/6(Out5) -> Out6/1
  Demux8_/2(Out1) -> Out2/1
  Demux8_/3(Out2) -> Out3/1
  Demux8_1/8(Out7) -> Out16/1
  Chan/1 -> msb_b_/1, lsb_ui3_/1
  lsb_ui3_/1 -> Demux8_1/1(Addr), Demux8_/1(Addr)
  msb_b_/1 -> Demux8_1/3(en), Inverter/1
  din/1 -> Demux8_1/2(BitIn), Demux8_/2(BitIn)
  Inverter/1 -> Demux8_/3(en)

== system fftanalyzeri/FIFO64_3/FIFO32_0/FIFO16Cir_1/CounterArray1/demux16_ ==
  Chan : Inport
  din : Inport  Port=2
  Demux8_ : Subsystem
  Demux8_1 : Subsystem
  Inverter : xbsIndex_r4/Inverter  en=off  latency=0  dbl_ovrd=off  block_type=inv
  lsb_ui3_ : xbsIndex_r4/Slice  nbits=3  boolean_output=off  mode=Lower Bit Location + Width  bit1=0  base1=MSB of Input  bit0=0  base0=LSB of Input  dbl_ovrd=off  block_type=slice
  msb_b_ : xbsIndex_r4/Slice  nbits=1  boolean_output=on  mode=Upper Bit Location + Width  bit1=0  base1=MSB of Input  bit0=0  base0=LSB of Input  dbl_ovrd=off  block_type=slice
  Out1 : Outport
  Out2 : Outport  Port=2
  Out3 : Outport  Port=3
  Out4 : Outport  Port=4
  Out5 : Outport  Port=5
  Out6 : Outport  Port=6
  Out7 : Outport  Port=7
  Out8 : Outport  Port=8
  Out9 : Outport  Port=9
  Out10 : Outport  Port=10
  Out11 : Outport  Port=11
  Out12 : Outport  Port=12
  Out13 : Outport  Port=13
  Out14 : Outport  Port=14
  Out15 : Outport  Port=15
  Out16 : Outport  Port=16
  wires:
  Demux8_1/1(Out0) -> Out9/1
  Demux8_1/6(Out5) -> Out14/1
  Demux8_/5(Out4) -> Out5/1
  Demux8_/7(Out6) -> Out7/1
  Demux8_1/2(Out1) -> Out10/1
  Demux8_1/3(Out2) -> Out11/1
  Demux8_/4(Out3) -> Out4/1
  Demux8_1/7(Out6) -> Out15/1
  Demux8_1/4(Out3) -> Out12/1
  Demux8_/8(Out7) -> Out8/1
  Demux8_/1(Out0) -> Out1/1
  Demux8_1/5(Out4) -> Out13/1
  Demux8_/6(Out5) -> Out6/1
  Demux8_/2(Out1) -> Out2/1
  Demux8_/3(Out2) -> Out3/1
  Demux8_1/8(Out7) -> Out16/1
  Chan/1 -> msb_b_/1, lsb_ui3_/1
  lsb_ui3_/1 -> Demux8_1/1(Addr), Demux8_/1(Addr)
  msb_b_/1 -> Demux8_1/3(en), Inverter/1
  din/1 -> Demux8_1/2(BitIn), Demux8_/2(BitIn)
  Inverter/1 -> Demux8_/3(en)

== system fftanalyzeri/FIFO64_3/FIFO32_0/FIFO16Cir_1/CounterArray2/demux16_ ==
  Chan : Inport
  din : Inport  Port=2
  Demux8_ : Subsystem
  Demux8_1 : Subsystem
  Inverter : xbsIndex_r4/Inverter  en=off  latency=0  dbl_ovrd=off  block_type=inv
  lsb_ui3_ : xbsIndex_r4/Slice  nbits=3  boolean_output=off  mode=Lower Bit Location + Width  bit1=0  base1=MSB of Input  bit0=0  base0=LSB of Input  dbl_ovrd=off  block_type=slice
  msb_b_ : xbsIndex_r4/Slice  nbits=1  boolean_output=on  mode=Upper Bit Location + Width  bit1=0  base1=MSB of Input  bit0=0  base0=LSB of Input  dbl_ovrd=off  block_type=slice
  Out1 : Outport
  Out2 : Outport  Port=2
  Out3 : Outport  Port=3
  Out4 : Outport  Port=4
  Out5 : Outport  Port=5
  Out6 : Outport  Port=6
  Out7 : Outport  Port=7
  Out8 : Outport  Port=8
  Out9 : Outport  Port=9
  Out10 : Outport  Port=10
  Out11 : Outport  Port=11
  Out12 : Outport  Port=12
  Out13 : Outport  Port=13
  Out14 : Outport  Port=14
  Out15 : Outport  Port=15
  Out16 : Outport  Port=16
  wires:
  Demux8_1/1(Out0) -> Out9/1
  Demux8_1/6(Out5) -> Out14/1
  Demux8_/5(Out4) -> Out5/1
  Demux8_/7(Out6) -> Out7/1
  Demux8_1/2(Out1) -> Out10/1
  Demux8_1/3(Out2) -> Out11/1
  Demux8_/4(Out3) -> Out4/1
  Demux8_1/7(Out6) -> Out15/1
  Demux8_1/4(Out3) -> Out12/1
  Demux8_/8(Out7) -> Out8/1
  Demux8_/1(Out0) -> Out1/1
  Demux8_1/5(Out4) -> Out13/1
  Demux8_/6(Out5) -> Out6/1
  Demux8_/2(Out1) -> Out2/1
  Demux8_/3(Out2) -> Out3/1
  Demux8_1/8(Out7) -> Out16/1
  Chan/1 -> msb_b_/1, lsb_ui3_/1
  lsb_ui3_/1 -> Demux8_1/1(Addr), Demux8_/1(Addr)
  msb_b_/1 -> Demux8_1/3(en), Inverter/1
  din/1 -> Demux8_1/2(BitIn), Demux8_/2(BitIn)
  Inverter/1 -> Demux8_/3(en)

== system fftanalyzeri/FIFO64_3/FIFO32_0/FIFO16Cir_2/CounterArray1/demux16_ ==
  Chan : Inport
  din : Inport  Port=2
  Demux8_ : Subsystem
  Demux8_1 : Subsystem
  Inverter : xbsIndex_r4/Inverter  en=off  latency=0  dbl_ovrd=off  block_type=inv
  lsb_ui3_ : xbsIndex_r4/Slice  nbits=3  boolean_output=off  mode=Lower Bit Location + Width  bit1=0  base1=MSB of Input  bit0=0  base0=LSB of Input  dbl_ovrd=off  block_type=slice
  msb_b_ : xbsIndex_r4/Slice  nbits=1  boolean_output=on  mode=Upper Bit Location + Width  bit1=0  base1=MSB of Input  bit0=0  base0=LSB of Input  dbl_ovrd=off  block_type=slice
  Out1 : Outport
  Out2 : Outport  Port=2
  Out3 : Outport  Port=3
  Out4 : Outport  Port=4
  Out5 : Outport  Port=5
  Out6 : Outport  Port=6
  Out7 : Outport  Port=7
  Out8 : Outport  Port=8
  Out9 : Outport  Port=9
  Out10 : Outport  Port=10
  Out11 : Outport  Port=11
  Out12 : Outport  Port=12
  Out13 : Outport  Port=13
  Out14 : Outport  Port=14
  Out15 : Outport  Port=15
  Out16 : Outport  Port=16
  wires:
  Demux8_1/1(Out0) -> Out9/1
  Demux8_1/6(Out5) -> Out14/1
  Demux8_/5(Out4) -> Out5/1
  Demux8_/7(Out6) -> Out7/1
  Demux8_1/2(Out1) -> Out10/1
  Demux8_1/3(Out2) -> Out11/1
  Demux8_/4(Out3) -> Out4/1
  Demux8_1/7(Out6) -> Out15/1
  Demux8_1/4(Out3) -> Out12/1
  Demux8_/8(Out7) -> Out8/1
  Demux8_/1(Out0) -> Out1/1
  Demux8_1/5(Out4) -> Out13/1
  Demux8_/6(Out5) -> Out6/1
  Demux8_/2(Out1) -> Out2/1
  Demux8_/3(Out2) -> Out3/1
  Demux8_1/8(Out7) -> Out16/1
  Chan/1 -> msb_b_/1, lsb_ui3_/1
  lsb_ui3_/1 -> Demux8_1/1(Addr), Demux8_/1(Addr)
  msb_b_/1 -> Demux8_1/3(en), Inverter/1
  din/1 -> Demux8_1/2(BitIn), Demux8_/2(BitIn)
  Inverter/1 -> Demux8_/3(en)

== system fftanalyzeri/FIFO64_3/FIFO32_0/FIFO16Cir_2/CounterArray2/demux16_ ==
  Chan : Inport
  din : Inport  Port=2
  Demux8_ : Subsystem
  Demux8_1 : Subsystem
  Inverter : xbsIndex_r4/Inverter  en=off  latency=0  dbl_ovrd=off  block_type=inv
  lsb_ui3_ : xbsIndex_r4/Slice  nbits=3  boolean_output=off  mode=Lower Bit Location + Width  bit1=0  base1=MSB of Input  bit0=0  base0=LSB of Input  dbl_ovrd=off  block_type=slice
  msb_b_ : xbsIndex_r4/Slice  nbits=1  boolean_output=on  mode=Upper Bit Location + Width  bit1=0  base1=MSB of Input  bit0=0  base0=LSB of Input  dbl_ovrd=off  block_type=slice
  Out1 : Outport
  Out2 : Outport  Port=2
  Out3 : Outport  Port=3
  Out4 : Outport  Port=4
  Out5 : Outport  Port=5
  Out6 : Outport  Port=6
  Out7 : Outport  Port=7
  Out8 : Outport  Port=8
  Out9 : Outport  Port=9
  Out10 : Outport  Port=10
  Out11 : Outport  Port=11
  Out12 : Outport  Port=12
  Out13 : Outport  Port=13
  Out14 : Outport  Port=14
  Out15 : Outport  Port=15
  Out16 : Outport  Port=16
  wires:
  Demux8_1/1(Out0) -> Out9/1
  Demux8_1/6(Out5) -> Out14/1
  Demux8_/5(Out4) -> Out5/1
  Demux8_/7(Out6) -> Out7/1
  Demux8_1/2(Out1) -> Out10/1
  Demux8_1/3(Out2) -> Out11/1
  Demux8_/4(Out3) -> Out4/1
  Demux8_1/7(Out6) -> Out15/1
  Demux8_1/4(Out3) -> Out12/1
  Demux8_/8(Out7) -> Out8/1
  Demux8_/1(Out0) -> Out1/1
  Demux8_1/5(Out4) -> Out13/1
  Demux8_/6(Out5) -> Out6/1
  Demux8_/2(Out1) -> Out2/1
  Demux8_/3(Out2) -> Out3/1
  Demux8_1/8(Out7) -> Out16/1
  Chan/1 -> msb_b_/1, lsb_ui3_/1
  lsb_ui3_/1 -> Demux8_1/1(Addr), Demux8_/1(Addr)
  msb_b_/1 -> Demux8_1/3(en), Inverter/1
  din/1 -> Demux8_1/2(BitIn), Demux8_/2(BitIn)
  Inverter/1 -> Demux8_/3(en)

== system fftanalyzeri/FIFO64_3/FIFO32_1/FIFO16Cir_1/CounterArray1/demux16_ ==
  Chan : Inport
  din : Inport  Port=2
  Demux8_ : Subsystem
  Demux8_1 : Subsystem
  Inverter : xbsIndex_r4/Inverter  en=off  latency=0  dbl_ovrd=off  block_type=inv
  lsb_ui3_ : xbsIndex_r4/Slice  nbits=3  boolean_output=off  mode=Lower Bit Location + Width  bit1=0  base1=MSB of Input  bit0=0  base0=LSB of Input  dbl_ovrd=off  block_type=slice
  msb_b_ : xbsIndex_r4/Slice  nbits=1  boolean_output=on  mode=Upper Bit Location + Width  bit1=0  base1=MSB of Input  bit0=0  base0=LSB of Input  dbl_ovrd=off  block_type=slice
  Out1 : Outport
  Out2 : Outport  Port=2
  Out3 : Outport  Port=3
  Out4 : Outport  Port=4
  Out5 : Outport  Port=5
  Out6 : Outport  Port=6
  Out7 : Outport  Port=7
  Out8 : Outport  Port=8
  Out9 : Outport  Port=9
  Out10 : Outport  Port=10
  Out11 : Outport  Port=11
  Out12 : Outport  Port=12
  Out13 : Outport  Port=13
  Out14 : Outport  Port=14
  Out15 : Outport  Port=15
  Out16 : Outport  Port=16
  wires:
  Demux8_1/1(Out0) -> Out9/1
  Demux8_1/6(Out5) -> Out14/1
  Demux8_/5(Out4) -> Out5/1
  Demux8_/7(Out6) -> Out7/1
  Demux8_1/2(Out1) -> Out10/1
  Demux8_1/3(Out2) -> Out11/1
  Demux8_/4(Out3) -> Out4/1
  Demux8_1/7(Out6) -> Out15/1
  Demux8_1/4(Out3) -> Out12/1
  Demux8_/8(Out7) -> Out8/1
  Demux8_/1(Out0) -> Out1/1
  Demux8_1/5(Out4) -> Out13/1
  Demux8_/6(Out5) -> Out6/1
  Demux8_/2(Out1) -> Out2/1
  Demux8_/3(Out2) -> Out3/1
  Demux8_1/8(Out7) -> Out16/1
  Chan/1 -> msb_b_/1, lsb_ui3_/1
  lsb_ui3_/1 -> Demux8_1/1(Addr), Demux8_/1(Addr)
  msb_b_/1 -> Demux8_1/3(en), Inverter/1
  din/1 -> Demux8_1/2(BitIn), Demux8_/2(BitIn)
  Inverter/1 -> Demux8_/3(en)

== system fftanalyzeri/FIFO64_3/FIFO32_1/FIFO16Cir_1/CounterArray2/demux16_ ==
  Chan : Inport
  din : Inport  Port=2
  Demux8_ : Subsystem
  Demux8_1 : Subsystem
  Inverter : xbsIndex_r4/Inverter  en=off  latency=0  dbl_ovrd=off  block_type=inv
  lsb_ui3_ : xbsIndex_r4/Slice  nbits=3  boolean_output=off  mode=Lower Bit Location + Width  bit1=0  base1=MSB of Input  bit0=0  base0=LSB of Input  dbl_ovrd=off  block_type=slice
  msb_b_ : xbsIndex_r4/Slice  nbits=1  boolean_output=on  mode=Upper Bit Location + Width  bit1=0  base1=MSB of Input  bit0=0  base0=LSB of Input  dbl_ovrd=off  block_type=slice
  Out1 : Outport
  Out2 : Outport  Port=2
  Out3 : Outport  Port=3
  Out4 : Outport  Port=4
  Out5 : Outport  Port=5
  Out6 : Outport  Port=6
  Out7 : Outport  Port=7
  Out8 : Outport  Port=8
  Out9 : Outport  Port=9
  Out10 : Outport  Port=10
  Out11 : Outport  Port=11
  Out12 : Outport  Port=12
  Out13 : Outport  Port=13
  Out14 : Outport  Port=14
  Out15 : Outport  Port=15
  Out16 : Outport  Port=16
  wires:
  Demux8_1/1(Out0) -> Out9/1
  Demux8_1/6(Out5) -> Out14/1
  Demux8_/5(Out4) -> Out5/1
  Demux8_/7(Out6) -> Out7/1
  Demux8_1/2(Out1) -> Out10/1
  Demux8_1/3(Out2) -> Out11/1
  Demux8_/4(Out3) -> Out4/1
  Demux8_1/7(Out6) -> Out15/1
  Demux8_1/4(Out3) -> Out12/1
  Demux8_/8(Out7) -> Out8/1
  Demux8_/1(Out0) -> Out1/1
  Demux8_1/5(Out4) -> Out13/1
  Demux8_/6(Out5) -> Out6/1
  Demux8_/2(Out1) -> Out2/1
  Demux8_/3(Out2) -> Out3/1
  Demux8_1/8(Out7) -> Out16/1
  Chan/1 -> msb_b_/1, lsb_ui3_/1
  lsb_ui3_/1 -> Demux8_1/1(Addr), Demux8_/1(Addr)
  msb_b_/1 -> Demux8_1/3(en), Inverter/1
  din/1 -> Demux8_1/2(BitIn), Demux8_/2(BitIn)
  Inverter/1 -> Demux8_/3(en)

== system fftanalyzeri/FIFO64_3/FIFO32_1/FIFO16Cir_2/CounterArray1/demux16_ ==
  Chan : Inport
  din : Inport  Port=2
  Demux8_ : Subsystem
  Demux8_1 : Subsystem
  Inverter : xbsIndex_r4/Inverter  en=off  latency=0  dbl_ovrd=off  block_type=inv
  lsb_ui3_ : xbsIndex_r4/Slice  nbits=3  boolean_output=off  mode=Lower Bit Location + Width  bit1=0  base1=MSB of Input  bit0=0  base0=LSB of Input  dbl_ovrd=off  block_type=slice
  msb_b_ : xbsIndex_r4/Slice  nbits=1  boolean_output=on  mode=Upper Bit Location + Width  bit1=0  base1=MSB of Input  bit0=0  base0=LSB of Input  dbl_ovrd=off  block_type=slice
  Out1 : Outport
  Out2 : Outport  Port=2
  Out3 : Outport  Port=3
  Out4 : Outport  Port=4
  Out5 : Outport  Port=5
  Out6 : Outport  Port=6
  Out7 : Outport  Port=7
  Out8 : Outport  Port=8
  Out9 : Outport  Port=9
  Out10 : Outport  Port=10
  Out11 : Outport  Port=11
  Out12 : Outport  Port=12
  Out13 : Outport  Port=13
  Out14 : Outport  Port=14
  Out15 : Outport  Port=15
  Out16 : Outport  Port=16
  wires:
  Demux8_1/1(Out0) -> Out9/1
  Demux8_1/6(Out5) -> Out14/1
  Demux8_/5(Out4) -> Out5/1
  Demux8_/7(Out6) -> Out7/1
  Demux8_1/2(Out1) -> Out10/1
  Demux8_1/3(Out2) -> Out11/1
  Demux8_/4(Out3) -> Out4/1
  Demux8_1/7(Out6) -> Out15/1
  Demux8_1/4(Out3) -> Out12/1
  Demux8_/8(Out7) -> Out8/1
  Demux8_/1(Out0) -> Out1/1
  Demux8_1/5(Out4) -> Out13/1
  Demux8_/6(Out5) -> Out6/1
  Demux8_/2(Out1) -> Out2/1
  Demux8_/3(Out2) -> Out3/1
  Demux8_1/8(Out7) -> Out16/1
  Chan/1 -> msb_b_/1, lsb_ui3_/1
  lsb_ui3_/1 -> Demux8_1/1(Addr), Demux8_/1(Addr)
  msb_b_/1 -> Demux8_1/3(en), Inverter/1
  din/1 -> Demux8_1/2(BitIn), Demux8_/2(BitIn)
  Inverter/1 -> Demux8_/3(en)

== system fftanalyzeri/FIFO64_3/FIFO32_1/FIFO16Cir_2/CounterArray2/demux16_ ==
  Chan : Inport
  din : Inport  Port=2
  Demux8_ : Subsystem
  Demux8_1 : Subsystem
  Inverter : xbsIndex_r4/Inverter  en=off  latency=0  dbl_ovrd=off  block_type=inv
  lsb_ui3_ : xbsIndex_r4/Slice  nbits=3  boolean_output=off  mode=Lower Bit Location + Width  bit1=0  base1=MSB of Input  bit0=0  base0=LSB of Input  dbl_ovrd=off  block_type=slice
  msb_b_ : xbsIndex_r4/Slice  nbits=1  boolean_output=on  mode=Upper Bit Location + Width  bit1=0  base1=MSB of Input  bit0=0  base0=LSB of Input  dbl_ovrd=off  block_type=slice
  Out1 : Outport
  Out2 : Outport  Port=2
  Out3 : Outport  Port=3
  Out4 : Outport  Port=4
  Out5 : Outport  Port=5
  Out6 : Outport  Port=6
  Out7 : Outport  Port=7
  Out8 : Outport  Port=8
  Out9 : Outport  Port=9
  Out10 : Outport  Port=10
  Out11 : Outport  Port=11
  Out12 : Outport  Port=12
  Out13 : Outport  Port=13
  Out14 : Outport  Port=14
  Out15 : Outport  Port=15
  Out16 : Outport  Port=16
  wires:
  Demux8_1/1(Out0) -> Out9/1
  Demux8_1/6(Out5) -> Out14/1
  Demux8_/5(Out4) -> Out5/1
  Demux8_/7(Out6) -> Out7/1
  Demux8_1/2(Out1) -> Out10/1
  Demux8_1/3(Out2) -> Out11/1
  Demux8_/4(Out3) -> Out4/1
  Demux8_1/7(Out6) -> Out15/1
  Demux8_1/4(Out3) -> Out12/1
  Demux8_/8(Out7) -> Out8/1
  Demux8_/1(Out0) -> Out1/1
  Demux8_1/5(Out4) -> Out13/1
  Demux8_/6(Out5) -> Out6/1
  Demux8_/2(Out1) -> Out2/1
  Demux8_/3(Out2) -> Out3/1
  Demux8_1/8(Out7) -> Out16/1
  Chan/1 -> msb_b_/1, lsb_ui3_/1
  lsb_ui3_/1 -> Demux8_1/1(Addr), Demux8_/1(Addr)
  msb_b_/1 -> Demux8_1/3(en), Inverter/1
  din/1 -> Demux8_1/2(BitIn), Demux8_/2(BitIn)
  Inverter/1 -> Demux8_/3(en)

== system fftanalyzeri/adcWaveMem/MemRecord/Shared BRAM/mem/calc_add ==
  note: Use behavioural HDL
      | so that gets optimised
      | to minimum logic
  note: If reading/writing words
      | smaller than 32 bits,
      | change address so
      | that addressing is
      | big endian instead of
      | little, otherwise
      | pass through
  in : Inport
  add_sub : xbsIndex_r4/AddSub  mode=Subtraction  use_carryin=off  use_carryout=off  en=off  latency=0  precision=User Defined  arith_type=Unsigned  n_bits=max(1, log2(32/data_width))  bin_pt=0  quantization=Truncate  overflow=Wrap  dbl_ovrd=off  use_behavioral_HDL=on  hw_selection=Fabric  pipelined=off  block_type=addsub
  concat : xbsIndex_r4/Concat  num_inputs=2  dbl_ovrd=off  block_type=concat
  const : xbsIndex_r4/Constant  const=max(0, 32/data_width-1)  gui_display_data_type=Fixed-point  arith_type=Unsigned  n_bits=max(1, log2(32/data_width))  bin_pt=0  preci_type=Single  exp_width=8  frac_width=24  explicit_period=on  period=sample_rate  equ=P=C  opselect=C  inp2=PCIN>>17  opr=+  inp1=P  carry=CIN  dbl_ovrd=off  block_type=constant
      settings: block_version=11.4
  convert_addr : xbsIndex_r4/Convert  gui_display_data_type=Fixed-point  arith_type=Unsigned  n_bits=addr_width  bin_pt=0  float_type=Single  exp_bits=8  fraction_bits=24  quantization=Truncate  overflow=Wrap  en=off  latency=0  dbl_ovrd=off  pipeline=off  block_type=convert
      settings: xl_area=[0, 0, 0, 0, 0, 0, 0]
  lsw : xbsIndex_r4/Slice  nbits=max(1, log2(32/data_width))  boolean_output=off  mode=Lower Bit Location + Width  bit1=0  base1=MSB of Input  bit0=0  base0=LSB of Input  dbl_ovrd=off  block_type=slice
  manipulate : xbsIndex_r4/Constant  const=min(1, floor(32/data_width) - 1)  gui_display_data_type=Fixed-point  arith_type=Unsigned  n_bits=1  bin_pt=0  preci_type=Single  exp_width=8  frac_width=24  explicit_period=on  period=sample_rate  equ=P=C  opselect=C  inp2=PCIN>>17  opr=+  inp1=P  carry=CIN  dbl_ovrd=off  block_type=constant
      settings: block_version=11.4
  msw : xbsIndex_r4/Slice  nbits=addr_width - max(1, log2(32/data_width))  boolean_output=off  mode=Upper Bit Location + Width  bit1=0  base1=MSB of Input  bit0=0  base0=LSB of Input  dbl_ovrd=off  block_type=slice
  mux : xbsIndex_r4/Mux  inputs=2  en=off  latency=0  precision=Full  arith_type=Unsigned  n_bits=16  bin_pt=14  quantization=Truncate  overflow=Wrap  dbl_ovrd=off  block_type=mux
      settings: block_version=11.4
  out : Outport
  wires:
  convert_addr/1 -> mux/2, msw/1, lsw/1
  const/1 -> add_sub/1
  lsw/1 -> add_sub/2
  mux/1 -> out/1
  manipulate/1 -> mux/1
  concat/1 -> mux/3
  msw/1 -> concat/1
  add_sub/1 -> concat/2
  in/1 -> convert_addr/1

== system fftanalyzeri/adcWaveMem/MemRecord/Shared BRAM/mem/sim_munge_in ==
  din : Inport
  reinterpret_out : xbsIndex_r4/Reinterpret  force_arith_type=on  arith_type=Unsigned  force_bin_pt=on  bin_pt=0  block_type=reinterpret
  dout : Outport
  wires:
  reinterpret_out/1 -> dout/1
  din/1 -> reinterpret_out/1

== system fftanalyzeri/adcWaveMem/MemRecord/Shared BRAM/mem/sim_munge_out ==
  din : Inport
  reinterpret_out : xbsIndex_r4/Reinterpret  force_arith_type=on  arith_type=Unsigned  force_bin_pt=on  bin_pt=0  block_type=reinterpret
  dout : Outport
  wires:
  reinterpret_out/1 -> dout/1
  din/1 -> reinterpret_out/1
